simulink model "intakeAirflow_var"  (R2018b)
settings: Solver=VariableStepAuto  StartTime=0.0  StopTime=10.0  RelTol=1e-3
model workspace (MAT data in the model file):
  PressVect = [0.05 0.1 0.15 0.2 0.25 0.3 0.35 0.4 0.45 0.5 0.55 0.6 0.65 0.7 0.75 0.8 0.85 0.9 0.95]
  PumpCon = [-0.0556348 -0.0022828 0.0256932 0.0435188 0.0562692 0.0661194857143 0.0741572 0.08697 0.0972452 0.106070342857 0.1139892 0.121303866667 ... (342 elements, 18x19)]
  RampRateKiX = [100 200 300 400 500 600]
  RampRateKiY = [0 0.2 0.4 0.6 0.8 1]
  RampRateKiZ = [0.012  0.024  0.036  0.048  0.06  0.072; 0.024  0.048  0.072  0.096  0.12  0.144; 0.036  0.072  0.108  0.144  0.18  0.216; 0.048  0.096  0.144  0.192  0.24  0.288; 0.06  0.12  0.18  0.24  0.3  0.36; 0.072  0.144  0.216  0.288  0.36  0.432]
  SpeedVect = [50 75 100 125 150 175 200 250 300 350 400 450 500 600 700 800 900 1000]
undefined symbols (not defined in the file or in its folder): sld_FuelModes
libraries: simulink x1
settings Model: Creator=rjongeli  LastModifiedBy=rjongeli
settings OptimizationCC: DefaultParameterBehavior=Inlined  UseDivisionForNetSlopeComputation=UseDivisionForReciprocalsOfIntegersOnly  InlineInvariantSignals=on  EnhancedBackFolding=on  StrengthReduction=on  BooleansAsBitfields=on  PassReuseOutputArgsAs=Individual arguments  ExpressionDepthLimit=2147483647  ZeroExternalMemoryAtStartup=off  ZeroInternalMemoryAtStartup=off  NoFixptDivByZeroProtection=on  EfficientFloat2IntCast=on  LifeSpan=1

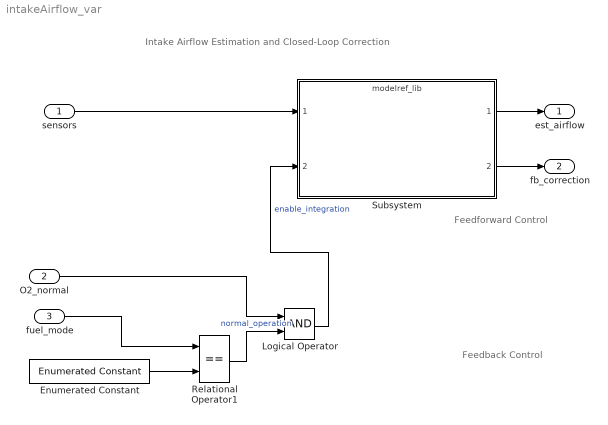
== system intakeAirflow_var ==
  note: Feedback Control
  note: Feedforward Control
  note: Intake Airflow Estimation and Closed-Loop Correction
  sensors : Inport  OutDataTypeStr=Bus: EngSensors
  O2_normal : Inport  Port=2
  fuel_mode : Inport  Port=3
  Enumerated Constant : simulink/Sources/Enumerated Constant  OutDataTypeStr=Enum: sld_FuelModes  Value=sld_FuelModes.LOW  SampleTime=.01
      settings: SourceProductName=Simulink
  Logical Operator : Logic  AllPortsSameDT=off  OutDataTypeStr=boolean
  Relational Operator1 : RelationalOperator  Operator===  OutDataTypeStr=boolean  RndMeth=Nearest  InputSameDT=on
  Subsystem : ModelReference  ModelNameDialog=modelref_lib  SimulationMode=Normal  ModelReferenceVersion=1.18
  est_airflow : Outport  Unit=g/s
  fb_correction : Outport  Port=2
  wires:
  Enumerated Constant/1 -> Relational Operator1/2
  Relational Operator1/1 -> Logical Operator/2  "normal_operation"
  fuel_mode/1 -> Relational Operator1/1
  O2_normal/1 -> Logical Operator/1
  sensors/1 -> Subsystem/1
  Logical Operator/1 -> Subsystem/2  "enable_integration"
  Subsystem/1 -> est_airflow/1
  Subsystem/2 -> fb_correction/1
